simulink model "untitled6"  (R2023b)
settings: Solver=VariableStepAuto  StartTime=0.0  StopTime=10.0  RelTol=1e-3
settings Model: Creator=A  LastModifiedBy=A

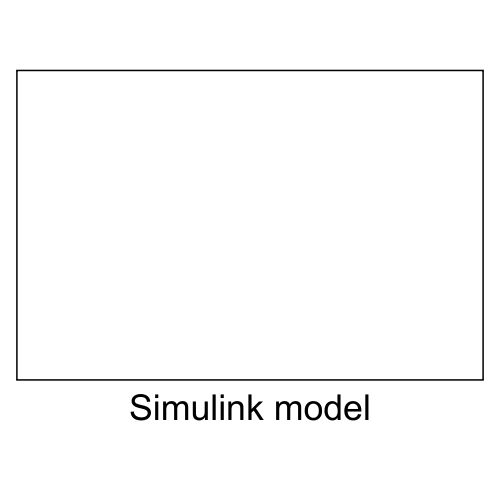
[thumbnail: Simulink's stored preview of the top-level diagram]
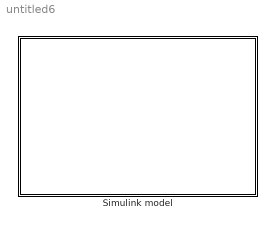
== system untitled6 ==
  Simulink model : Subsystem

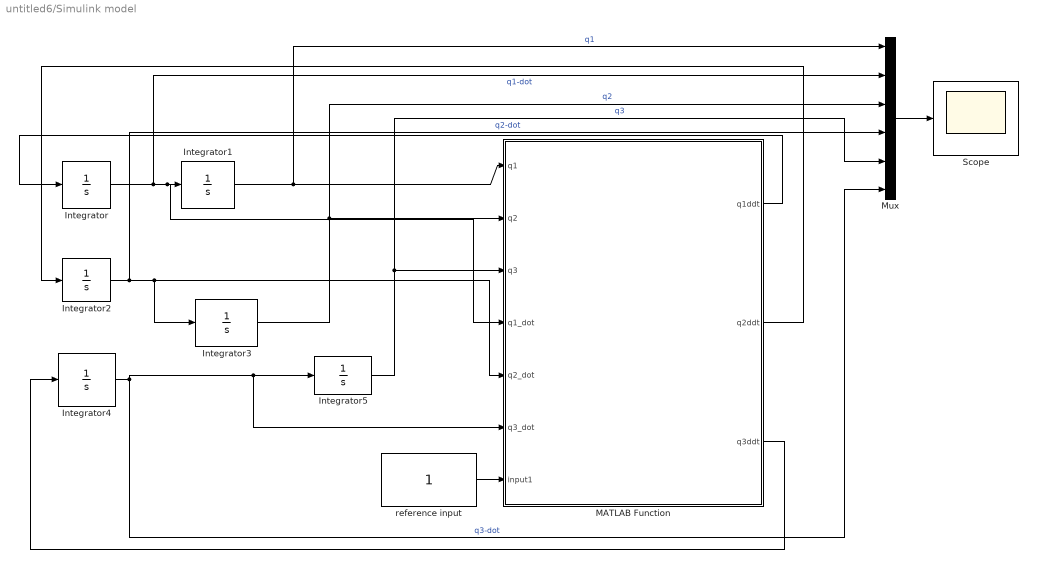
== system untitled6/Simulink model ==
  Integrator{,1..5} (6 alike) : Integrator
  MATLAB Function : MATLAB Function  TreatAsAtomicUnit=on
  Mux : Mux  Inputs=6
  Scope : Scope
  reference input : Constant
  wires:
  Integrator4/1 -> Mux/6, Integrator5/1, MATLAB Function/6(q3_dot)  "q3-dot"
  Integrator1/1 -> Mux/1, MATLAB Function/1(q1)  "q1"
  MATLAB Function/2(q2ddt) -> Integrator2/1
  MATLAB Function/1(q1ddt) -> Integrator/1
  Integrator2/1 -> Mux/4, Integrator3/1, MATLAB Function/5(q2_dot)  "q2-dot"
  Integrator/1 -> Mux/2, MATLAB Function/4(q1_dot), Integrator1/1  "q1-dot"
  MATLAB Function/3(q3ddt) -> Integrator4/1
  Integrator3/1 -> Mux/3, MATLAB Function/2(q2)  "q2"
  Integrator5/1 -> Mux/5, MATLAB Function/3(q3)  "q3"
  reference input/1 -> MATLAB Function/7(input1)
  Mux/1 -> Scope/1

== matlab function untitled6/Simulink model/MATLAB Function ==
  data: q1 input; q1ddt output; q2 input; q3 input; q1_dot input; q2_dot input; q3_dot input; q2ddt output; q3ddt output; input1 input
function [q1ddt,q2ddt,q3ddt] = fcn(q1,q2,q3,q1_dot,q2_dot,q3_dot, input1)

I1=(m1/12)*L1*L1;
I2=(m2/12)*L2*L2;
I3=(m3/12)*L3*L3;

d11=I1 + I2/2 + I3/2 - (I3*cos(2*x2 + 2*x3))/2 + (L1^2*m1)/4 + L1^2*m2 + L1^2*m3 + (L2^2*m2)/8 + (L2^2*m3)/2 + (L3^2*m3)/8 - (I2*cos(2*x2))/2 - (L2^2*m2*cos(2*x2))/8 - (L2^2*m3*cos(2*x2))/2 - (L3^2*m3*cos(2*x2 + 2*x3))/8 + (L2*L3*m3*cos(x3))/2 - (L2*L3*m3*cos(2*x2 + x3))/2;
d12=-(L1*(L3*m3*cos(x2 + x3) + L2*m2*cos(x2) + 2*L2*m3*cos(x2)))/2;
d13=-(L1*L3*m3*cos(x2 + x3))/2;
d21=d12;
d22=I2 + I3 + (L2^2*m2)/4 + L2^2*m3 + (L3^2*m3)/4 + L2*L3*m3*cos(x3);
d23=(m3*L3^2)/4 + (L2*m3*cos(x3)*L3)/2 + I3;
d31=d13;
d32=d23;
d33=(m3*L3^2)/4 + I3;
Dq=[d11,d12,d13;
    d21,d22,d23;
    d31,d32,d33];


c11=I3*x1_dot*x2_dot*sin(2*x2 + 2*x3) + I3*x1_dot*x3_dot*sin(2*x2 + 2*x3) + I2*x1_dot*x2_dot*sin(2*x2) + (L1*L2*m2*x2_dot^2*sin(x2))/2 + L1*L2*m3*x2_dot^2*sin(x2) + (L2^2*m2*x1_dot*x2_dot*sin(2*x2))/4 + L2^2*m3*x1_dot*x2_dot*sin(2*x2) + (L3^2*m3*x1_dot*x2_dot*sin(2*x2 + 2*x3))/4 + (L3^2*m3*x1_dot*x3_dot*sin(2*x2 + 2*x3))/4 + (L1*L3*m3*x2_dot^2*sin(x2 + x3))/2 + (L1*L3*m3*x3_dot^2*sin(x2 + x3))/2 + L1*L3*m3*x2_dot*x3_dot*sin(x2 + x3) - (L2*L3*m3*x1_dot*x3_dot*sin(x3))/2 + L2*L3*m3*x1_dot*x2_dot*sin(2*x2 + x3) + (L2*L3*m3*x1_dot*x3_dot*sin(2*x2 + x3))/2;
c21= -(I3*x1_dot^2*sin(2*x2 + 2*x3))/2 - (I2*x1_dot^2*sin(2*x2))/2 - (L2^2*m2*x1_dot^2*sin(2*x2))/8 - (L2^2*m3*x1_dot^2*sin(2*x2))/2 - (L3^2*m3*x1_dot^2*sin(2*x2 + 2*x3))/8 - (L2*L3*m3*x3_dot^2*sin(x3))/2 - (L2*L3*m3*x1_dot^2*sin(2*x2 + x3))/2 - L2*L3*m3*x2_dot*x3_dot*sin(x3);
c31= ((L2*L3*m3*sin(x3))/4 - (L3^2*m3*sin(2*x2 + 2*x3))/8 - (I3*sin(2*x2 + 2*x3))/2 - (L2*L3*m3*sin(2*x2 + x3))/4)*x1_dot^2 + (L2*L3*m3*sin(x3)*x2_dot^2)/2;
cq=[c11;
    c21;
    c31];

g11=0;
g21=- g*m3*((L3*sin(x2 + x3))/2 + L2*sin(x2)) - (L2*g*m2*sin(x2))/2;
g31=-(L3*g*m3*sin(x2 + x3))/2;
Gq=[g11;
    g21;
    g31];

W11=C1*x1_dot;
W21=C2*x2_dot;
W31=C3*x3_dot;
Fi=[W11;
    W21;
    W31];

tau=[tau1;
    0;
    0];

ddx = Dq \ (tau - cq - Gq - Fi);
x1ddt=ddx(1,:);
x2ddt=ddx(2,:);
x3ddt=ddx(3,:);
